simulink model "atrias_system_1khz"  (R2016b)
settings: Solver=FixedStepDiscrete  StartTime=0.0  StopTime=inf  FixedStep=sample_time  RelTol=1e-3
undefined symbols (not defined in the file or in its folder): gui_disable_cmd, gui_enable_cmd, gui_exit_cmd, gui_reset_cmd, HARD_MOTOR_POSITION_LIMITS_LOWER, HARD_MOTOR_POSITION_LIMITS_UPPER, HIP_ABS_MAX_ENCODER_TICKS, HIP_CURRENT_LIMIT, HIP_INC_MAX_ENCODER_TICKS, HIP_MOTOR_CONSTANT, HIP_MTR_GEAR_RATIO, HIP_MTR_MAX_TORQUE, LEFT_MOTOR_HIP_DIRECTION, LEG1_MOTOR_A_DIRECTION, LEG1_MOTOR_B_DIRECTION, LEG2_MOTOR_A_DIRECTION, LEG2_MOTOR_B_DIRECTION, LEG_CURRENT_LIMIT, LEG_INC_ENCODER_DIRECTION_LEFT_BACK, LEG_INC_ENCODER_DIRECTION_LEFT_FRONT, LEG_INC_ENCODER_DIRECTION_RIGHT_BACK, LEG_INC_ENCODER_DIRECTION_RIGHT_FRONT, LEG_INC_ENCODER_RAD_PER_TICK, LEG_MOTOR_CONSTANT, LEG_MTR_GEAR_RATIO, LEG_MTR_MAX_TORQUE, max_hip_velocity, max_motor_velocity, MEDULLA_ADC_MAX_VOLTS, MEDULLA_ADC_OFFSET_COUNTS, MEDULLA_STATE_ERROR, MEDULLA_STATE_HALT, MEDULLA_STATE_IDLE, MEDULLA_STATE_RESET, MEDULLA_STATE_RUN, MOTOR_POSITION_LIMITS_LOWER, MOTOR_POSITION_LIMITS_UPPER, MTR_HIP_MAX_CURRENT, MTR_MAX_CONT_CURRENT, MTR_MAX_COUNT, MTR_MAX_CURRENT, MTR_MAX_TEMP, RIGHT_MOTOR_HIP_DIRECTION
libraries: xpcethercatlib x190, simulink x37
(part 3 of 4)

== system atrias_system_1khz/DAQ/Conversion ==
  note: Convert from Current to Torque
  Elmo Current : Inport
  Constant10 : Constant  Value=LEG_MOTOR_CONSTANT
  Constant11 : Constant  Value=LEG_MTR_GEAR_RATIO
  Convert Elmo PDO to Current : Gain  Gain=MTR_MAX_CONT_CURRENT/1000
  Divide2 : Product  Inputs=****
  LEG1_MOTOR_A_DIRECTION : Constant  Value=LEG1_MOTOR_A_DIRECTION
  LEG1_MOTOR_B_DIRECTION : Constant  Value=LEG1_MOTOR_B_DIRECTION
  LEG2_MOTOR_A_DIRECTION : Constant  Value=LEG2_MOTOR_A_DIRECTION
  LEG2_MOTOR_B_DIRECTION : Constant  Value=LEG2_MOTOR_B_DIRECTION
  Mux2 : Mux
  Torque : Outport
  wires:
  Elmo Current/1 -> Convert Elmo PDO to Current/1
  Constant11/1 -> Divide2/2
  Convert Elmo PDO to Current/1 -> Divide2/3
  Constant10/1 -> Divide2/1
  Divide2/1 -> Torque/1
  LEG1_MOTOR_A_DIRECTION/1 -> Mux2/1
  LEG2_MOTOR_B_DIRECTION/1 -> Mux2/4
  Mux2/1 -> Divide2/4
  LEG2_MOTOR_A_DIRECTION/1 -> Mux2/3
  LEG1_MOTOR_B_DIRECTION/1 -> Mux2/2

== system atrias_system_1khz/DAQ/Conversion1 ==
  note: Convert from Current to Torque
  Elmo Current : Inport
  Constant10 : Constant  Value=LEG_MOTOR_CONSTANT
  Constant11 : Constant  Value=LEG_MTR_GEAR_RATIO
  Convert Elmo PDO to Current : Gain  Gain=MTR_MAX_CONT_CURRENT/1000
  Divide2 : Product  Inputs=****
  LEG1_MOTOR_A_DIRECTION : Constant  Value=LEG1_MOTOR_A_DIRECTION
  LEG1_MOTOR_B_DIRECTION : Constant  Value=LEG1_MOTOR_B_DIRECTION
  LEG2_MOTOR_A_DIRECTION : Constant  Value=LEG2_MOTOR_A_DIRECTION
  LEG2_MOTOR_B_DIRECTION : Constant  Value=LEG2_MOTOR_B_DIRECTION
  Mux2 : Mux
  Torque : Outport
  wires:
  LEG1_MOTOR_B_DIRECTION/1 -> Mux2/2
  LEG2_MOTOR_A_DIRECTION/1 -> Mux2/3
  Mux2/1 -> Divide2/4
  LEG2_MOTOR_B_DIRECTION/1 -> Mux2/4
  LEG1_MOTOR_A_DIRECTION/1 -> Mux2/1
  Divide2/1 -> Torque/1
  Constant10/1 -> Divide2/1
  Convert Elmo PDO to Current/1 -> Divide2/3
  Constant11/1 -> Divide2/2
  Elmo Current/1 -> Convert Elmo PDO to Current/1

== system atrias_system_1khz/DAQ/Convert geared rad//s to rotor cnts//s ==
  in : Inport
  Gear Ratio : Gain  Gain=LEG_MTR_GEAR_RATIO
  LEG1_MOTOR_A_DIRECTION : Constant  Value=LEG1_MOTOR_A_DIRECTION
  LEG1_MOTOR_B_DIRECTION : Constant  Value=LEG1_MOTOR_B_DIRECTION
  LEG2_MOTOR_A_DIRECTION : Constant  Value=LEG2_MOTOR_A_DIRECTION
  LEG2_MOTOR_B_DIRECTION : Constant  Value=LEG2_MOTOR_B_DIRECTION
  Mux2 : Mux
  Product : Product  RndMeth=Zero
  RadPerSecToCountsPerSec : Gain  Gain=14000/(2*pi)
  out : Outport
  wires:
  RadPerSecToCountsPerSec/1 -> Gear Ratio/1
  in/1 -> RadPerSecToCountsPerSec/1
  LEG1_MOTOR_A_DIRECTION/1 -> Mux2/1
  Product/1 -> out/1
  Gear Ratio/1 -> Product/1
  LEG2_MOTOR_B_DIRECTION/1 -> Mux2/4
  Mux2/1 -> Product/2
  LEG2_MOTOR_A_DIRECTION/1 -> Mux2/3
  LEG1_MOTOR_B_DIRECTION/1 -> Mux2/2

== system atrias_system_1khz/DAQ/Convert rotor cnt//s to geared rad//s ==
  in : Inport
  Divide : Product  Inputs=*//
  Gear Ratio : Gain  Gain=LEG_MTR_GEAR_RATIO
  LEG1_MOTOR_A_DIRECTION : Constant  Value=LEG1_MOTOR_A_DIRECTION
  LEG1_MOTOR_B_DIRECTION : Constant  Value=LEG1_MOTOR_B_DIRECTION
  LEG2_MOTOR_A_DIRECTION : Constant  Value=LEG2_MOTOR_A_DIRECTION
  LEG2_MOTOR_B_DIRECTION : Constant  Value=LEG2_MOTOR_B_DIRECTION
  Mux : Mux  Inputs=2
  Mux2 : Mux
  RadPerSecToCountsPerSec : Constant  Value=14000/(2*pi)
  out : Outport
  wires:
  RadPerSecToCountsPerSec/1 -> Gear Ratio/1
  in/1 -> Divide/1
  LEG1_MOTOR_A_DIRECTION/1 -> Mux2/1
  Divide/1 -> out/1
  Gear Ratio/1 -> Divide/2
  LEG2_MOTOR_B_DIRECTION/1 -> Mux2/4
  Mux2/1 -> Mux/1, Mux/2
  LEG2_MOTOR_A_DIRECTION/1 -> Mux2/3
  LEG1_MOTOR_B_DIRECTION/1 -> Mux2/2
  Mux/1 -> Divide/3

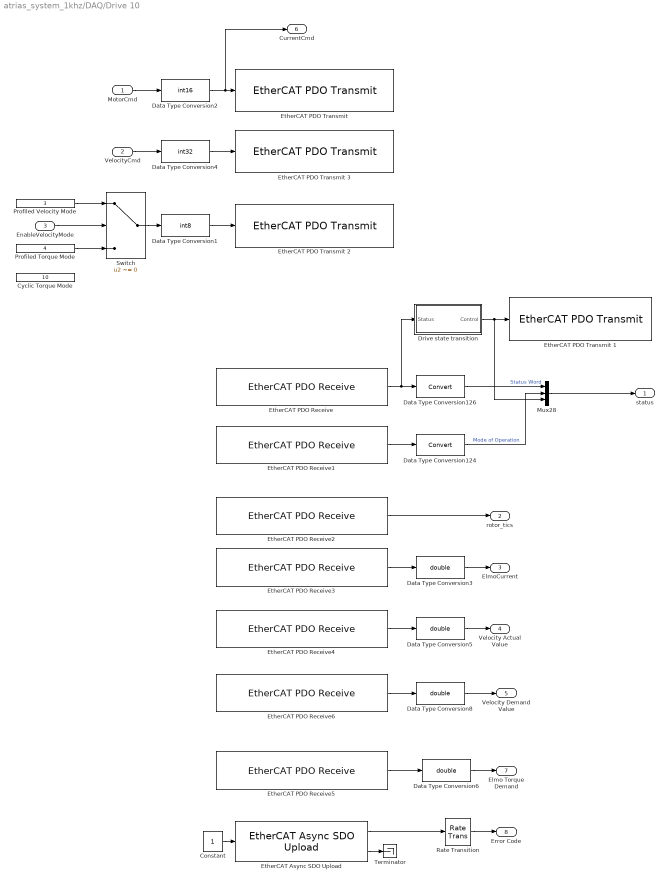
== system atrias_system_1khz/DAQ/Drive 10 ==
  MotorCmd : Inport
  VelocityCmd : Inport  Port=2
  EnableVelocityMode : Inport  Port=3
  Constant : Constant  OutDataTypeStr=int32
  Cyclic Torque Mode : Constant  Value=10  OutDataTypeStr=Inherit: Inherit via back propagation
  Data Type Conversion1 : DataTypeConversion  OutDataTypeStr=int8
  Data Type Conversion124 : DataTypeConversion
  Data Type Conversion126 : DataTypeConversion
  Data Type Conversion2 : DataTypeConversion  OutDataTypeStr=int16
  Data Type Conversion{3,5..6,8} (4 alike) : DataTypeConversion  OutDataTypeStr=double
  Data Type Conversion4 : DataTypeConversion  OutDataTypeStr=int32
  Drive state transition : Subsystem
  EtherCAT Async SDO Upload : xpcethercatlib/EtherCAT Async SDO Upload  index=24639  subIndex=0  sig_type=uint16  sig_dim=1  device_id=0  slave_name=Drive 10 (Elmo Drive)  sample_time=0.100  slave_addr=1010  selected_slave=Term 1 (EK1100)  timeout=500  slave_found=1
  EtherCAT PDO Receive : xpcethercatlib/EtherCAT PDO Receive  Priority=2  sig_name=Drive 10 (Elmo Drive).Inputs.Status word  sig_offset=3296  sig_type=uint16  type_size=16  sig_dim=1  device_id=0  sample_time=0.001000
  EtherCAT PDO Receive1 : xpcethercatlib/EtherCAT PDO Receive  Priority=2  sig_name=Drive 10 (Elmo Drive).Inputs.Mode of operation display  sig_offset=3312  sig_type=int8  type_size=8  sig_dim=1  device_id=0  sample_time=0.001000
  EtherCAT PDO Receive2 : xpcethercatlib/EtherCAT PDO Receive  Priority=2  sig_name=Drive 10 (Elmo Drive).Inputs.Position actual value  sig_offset=3328  sig_type=int32  type_size=32  sig_dim=1  device_id=0  sample_time=0.001000
  EtherCAT PDO Receive3 : xpcethercatlib/EtherCAT PDO Receive  Priority=2  sig_name=Drive 10 (Elmo Drive).Inputs.Current actual value  sig_offset=3440  sig_type=int16  type_size=16  sig_dim=1  device_id=0  sample_time=0.001000
  EtherCAT PDO Receive4 : xpcethercatlib/EtherCAT PDO Receive  Priority=2  sig_name=Drive 10 (Elmo Drive).Inputs.Velocity actual value  sig_offset=3392  sig_type=int32  type_size=32  sig_dim=1  device_id=0  sample_time=0.001000
  EtherCAT PDO Receive5 : xpcethercatlib/EtherCAT PDO Receive  Priority=2  sig_name=Drive 10 (Elmo Drive).Inputs.Torque demand value  sig_offset=3424  sig_type=int16  type_size=16  sig_dim=1  device_id=0  sample_time=0.001000
  EtherCAT PDO Receive6 : xpcethercatlib/EtherCAT PDO Receive  Priority=2  sig_name=Drive 10 (Elmo Drive).Inputs.Velocity demand [cnt/sec]  sig_offset=3360  sig_type=int32  type_size=32  sig_dim=1  device_id=0  sample_time=0.001000
  "EtherCAT PDO Transmit " : xpcethercatlib/EtherCAT PDO Transmit   Priority=3  sig_name=Drive 10 (Elmo Drive).Outputs.Target Torque  sig_offset=3328  sig_type=int16  type_size=16  sig_dim=1  device_id=0  sample_time=0.001000
  EtherCAT PDO Transmit 1 : xpcethercatlib/EtherCAT PDO Transmit   Priority=3  sig_name=Drive 10 (Elmo Drive).Outputs.Control word  sig_offset=3296  sig_type=uint16  type_size=16  sig_dim=1  device_id=0  sample_time=0.001000
  EtherCAT PDO Transmit 2 : xpcethercatlib/EtherCAT PDO Transmit   Priority=3  sig_name=Drive 10 (Elmo Drive).Outputs.Mode of operation  sig_offset=3312  sig_type=int8  type_size=8  sig_dim=1  device_id=0  sample_time=0.001000
  EtherCAT PDO Transmit 3 : xpcethercatlib/EtherCAT PDO Transmit   Priority=3  sig_name=Drive 10 (Elmo Drive).Outputs.Target Velocity  sig_offset=3360  sig_type=int32  type_size=32  sig_dim=1  device_id=0  sample_time=0.001000
  Mux28 : Mux  Inputs=3
  Profiled Torque Mode : Constant  Value=4  OutDataTypeStr=Inherit: Inherit via back propagation
  Profiled Velocity Mode : Constant  Value=3  OutDataTypeStr=Inherit: Inherit via back propagation
  Rate Transition : RateTransition  Deterministic=off  OutPortSampleTime=sample_time
  Switch : Switch  Criteria=u2 ~= 0
  Terminator : Terminator
  status : Outport
  rotor_tics : Outport  Port=2
  ElmoCurrent : Outport  Port=3
  Velocity Actual Value : Outport  Port=4
  Velocity Demand Value : Outport  Port=5
  CurrentCmd : Outport  Port=6
  Elmo Torque Demand : Outport  Port=7
  Error Code : Outport  Port=8
  wires:
  Data Type Conversion3/1 -> ElmoCurrent/1
  EtherCAT PDO Receive3/1 -> Data Type Conversion3/1
  EtherCAT PDO Receive2/1 -> rotor_tics/1
  Data Type Conversion2/1 -> CurrentCmd/1, "EtherCAT PDO Transmit "/1
  MotorCmd/1 -> Data Type Conversion2/1
  Data Type Conversion1/1 -> EtherCAT PDO Transmit 2/1
  Drive state transition/1(Control) -> EtherCAT PDO Transmit 1/1, Mux28/3
  Switch/1 -> Data Type Conversion1/1
  Data Type Conversion124/1 -> Mux28/2  "Mode of Operation"
  Data Type Conversion126/1 -> Mux28/1  "Status Word"
  Mux28/1 -> status/1
  EtherCAT PDO Receive1/1 -> Data Type Conversion124/1
  EtherCAT PDO Receive/1 -> Drive state transition/1(Status), Data Type Conversion126/1
  Profiled Torque Mode/1 -> Switch/3
  Profiled Velocity Mode/1 -> Switch/1
  EnableVelocityMode/1 -> Switch/2
  Data Type Conversion4/1 -> EtherCAT PDO Transmit 3/1
  VelocityCmd/1 -> Data Type Conversion4/1
  EtherCAT PDO Receive4/1 -> Data Type Conversion5/1
  Data Type Conversion5/1 -> Velocity Actual Value/1
  Data Type Conversion6/1 -> Elmo Torque Demand/1
  EtherCAT PDO Receive5/1 -> Data Type Conversion6/1
  EtherCAT Async SDO Upload/1 -> Rate Transition/1
  Constant/1 -> EtherCAT Async SDO Upload/1
  Rate Transition/1 -> Error Code/1
  EtherCAT Async SDO Upload/2 -> Terminator/1
  EtherCAT PDO Receive6/1 -> Data Type Conversion8/1
  Data Type Conversion8/1 -> Velocity Demand Value/1

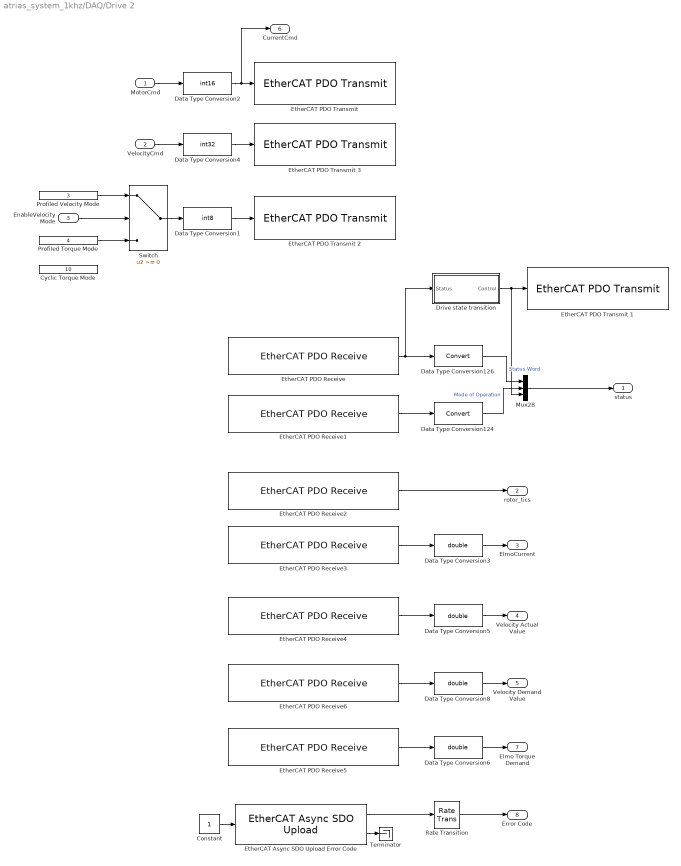
== system atrias_system_1khz/DAQ/Drive 2 ==
  MotorCmd : Inport
  VelocityCmd : Inport  Port=2
  EnableVelocity Mode : Inport  Port=3
  Constant : Constant  OutDataTypeStr=int32
  Cyclic Torque Mode : Constant  Value=10  OutDataTypeStr=Inherit: Inherit via back propagation
  Data Type Conversion1 : DataTypeConversion  OutDataTypeStr=int8
  Data Type Conversion124 : DataTypeConversion
  Data Type Conversion126 : DataTypeConversion
  Data Type Conversion2 : DataTypeConversion  OutDataTypeStr=int16
  Data Type Conversion{3,5..6,8} (4 alike) : DataTypeConversion  OutDataTypeStr=double
  Data Type Conversion4 : DataTypeConversion  OutDataTypeStr=int32
  Drive state transition : Subsystem
  EtherCAT Async SDO Upload Error Code : xpcethercatlib/EtherCAT Async SDO Upload  index=24639  subIndex=0  sig_type=uint16  sig_dim=1  device_id=0  slave_name=Box 2 (Elmo Drive)  sample_time=0.100  slave_addr=1002  selected_slave=Term 1 (EK1100)  timeout=500  slave_found=1
  EtherCAT PDO Receive : xpcethercatlib/EtherCAT PDO Receive  Priority=2  sig_name=Box 2 (Elmo Drive).Inputs.Status word  sig_offset=2816  sig_type=uint16  type_size=16  sig_dim=1  device_id=0  sample_time=0.001000
  EtherCAT PDO Receive1 : xpcethercatlib/EtherCAT PDO Receive  Priority=2  sig_name=Box 2 (Elmo Drive).Inputs.Mode of operation display  sig_offset=2832  sig_type=int8  type_size=8  sig_dim=1  device_id=0  sample_time=0.001000
  EtherCAT PDO Receive2 : xpcethercatlib/EtherCAT PDO Receive  Priority=2  sig_name=Box 2 (Elmo Drive).Inputs.Position actual value  sig_offset=2848  sig_type=int32  type_size=32  sig_dim=1  device_id=0  sample_time=0.001000
  EtherCAT PDO Receive3 : xpcethercatlib/EtherCAT PDO Receive  Priority=2  sig_name=Box 2 (Elmo Drive).Inputs.Current actual value  sig_offset=2960  sig_type=int16  type_size=16  sig_dim=1  device_id=0  sample_time=0.001000
  EtherCAT PDO Receive4 : xpcethercatlib/EtherCAT PDO Receive  Priority=2  sig_name=Box 2 (Elmo Drive).Inputs.Velocity actual value  sig_offset=2912  sig_type=int32  type_size=32  sig_dim=1  device_id=0  sample_time=0.001000
  EtherCAT PDO Receive5 : xpcethercatlib/EtherCAT PDO Receive  Priority=2  sig_name=Box 2 (Elmo Drive).Inputs.Torque demand value  sig_offset=2944  sig_type=int16  type_size=16  sig_dim=1  device_id=0  sample_time=0.001000
  EtherCAT PDO Receive6 : xpcethercatlib/EtherCAT PDO Receive  Priority=2  sig_name=Box 2 (Elmo Drive).Inputs.Velocity demand [cnt/sec]  sig_offset=2880  sig_type=int32  type_size=32  sig_dim=1  device_id=0  sample_time=0.001000
  "EtherCAT PDO Transmit " : xpcethercatlib/EtherCAT PDO Transmit   Priority=3  sig_name=Box 2 (Elmo Drive).Outputs.Target Torque  sig_offset=2848  sig_type=int16  type_size=16  sig_dim=1  device_id=0  sample_time=0.001000
  EtherCAT PDO Transmit 1 : xpcethercatlib/EtherCAT PDO Transmit   Priority=3  sig_name=Box 2 (Elmo Drive).Outputs.Control word  sig_offset=2816  sig_type=uint16  type_size=16  sig_dim=1  device_id=0  sample_time=0.001000
  EtherCAT PDO Transmit 2 : xpcethercatlib/EtherCAT PDO Transmit   Priority=3  sig_name=Box 2 (Elmo Drive).Outputs.Mode of operation  sig_offset=2832  sig_type=int8  type_size=8  sig_dim=1  device_id=0  sample_time=0.001000
  EtherCAT PDO Transmit 3 : xpcethercatlib/EtherCAT PDO Transmit   Priority=3  sig_name=Box 2 (Elmo Drive).Outputs.Target Velocity  sig_offset=2880  sig_type=int32  type_size=32  sig_dim=1  device_id=0  sample_time=0.001000
  Mux28 : Mux  Inputs=3
  Profiled Torque Mode : Constant  Value=4  OutDataTypeStr=Inherit: Inherit via back propagation
  Profiled Velocity Mode : Constant  Value=3  OutDataTypeStr=Inherit: Inherit via back propagation
  Rate Transition : RateTransition  Deterministic=off  OutPortSampleTime=sample_time
  Switch : Switch  Criteria=u2 ~= 0
  Terminator : Terminator
  status : Outport
  rotor_tics : Outport  Port=2
  ElmoCurrent : Outport  Port=3
  Velocity Actual Value : Outport  Port=4
  Velocity Demand Value : Outport  Port=5
  CurrentCmd : Outport  Port=6
  Elmo Torque Demand : Outport  Port=7
  Error Code : Outport  Port=8
  wires:
  EtherCAT PDO Receive1/1 -> Data Type Conversion124/1
  Mux28/1 -> status/1
  Data Type Conversion126/1 -> Mux28/1  "Status Word"
  Data Type Conversion124/1 -> Mux28/2  "Mode of Operation"
  Drive state transition/1(Control) -> Mux28/3, EtherCAT PDO Transmit 1/1
  EtherCAT PDO Receive2/1 -> rotor_tics/1
  EtherCAT PDO Receive3/1 -> Data Type Conversion3/1
  Data Type Conversion3/1 -> ElmoCurrent/1
  Data Type Conversion2/1 -> CurrentCmd/1, "EtherCAT PDO Transmit "/1
  MotorCmd/1 -> Data Type Conversion2/1
  Data Type Conversion1/1 -> EtherCAT PDO Transmit 2/1
  Switch/1 -> Data Type Conversion1/1
  Profiled Torque Mode/1 -> Switch/3
  Profiled Velocity Mode/1 -> Switch/1
  EnableVelocity Mode/1 -> Switch/2
  VelocityCmd/1 -> Data Type Conversion4/1
  Data Type Conversion4/1 -> EtherCAT PDO Transmit 3/1
  EtherCAT PDO Receive4/1 -> Data Type Conversion5/1
  Data Type Conversion5/1 -> Velocity Actual Value/1
  EtherCAT PDO Receive/1 -> Data Type Conversion126/1, Drive state transition/1(Status)
  Data Type Conversion6/1 -> Elmo Torque Demand/1
  EtherCAT PDO Receive5/1 -> Data Type Conversion6/1
  EtherCAT Async SDO Upload Error Code/1 -> Rate Transition/1
  Constant/1 -> EtherCAT Async SDO Upload Error Code/1
  Rate Transition/1 -> Error Code/1
  EtherCAT Async SDO Upload Error Code/2 -> Terminator/1
  EtherCAT PDO Receive6/1 -> Data Type Conversion8/1
  Data Type Conversion8/1 -> Velocity Demand Value/1

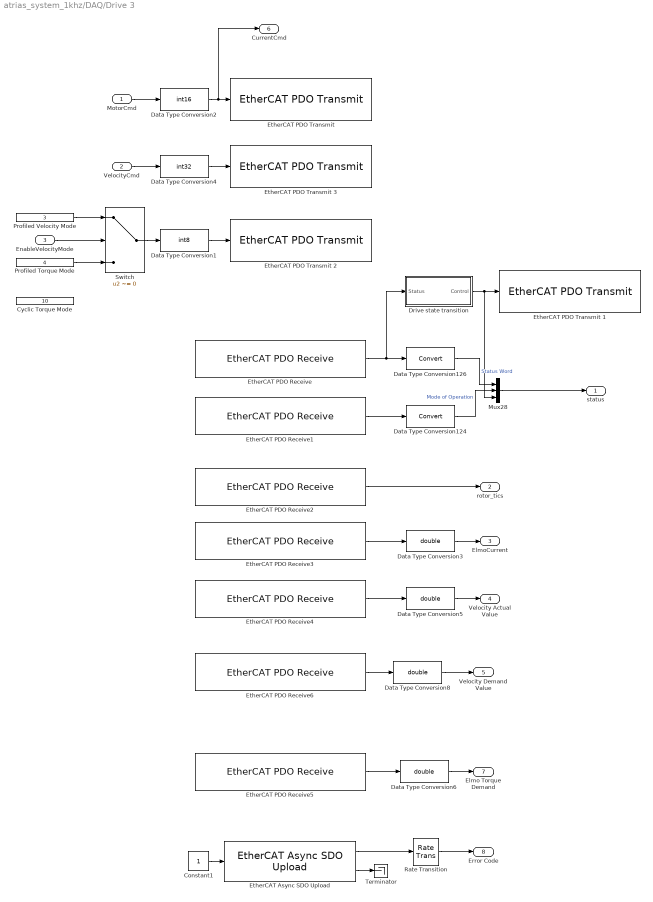
== system atrias_system_1khz/DAQ/Drive 3 ==
  MotorCmd : Inport
  VelocityCmd : Inport  Port=2
  EnableVelocityMode : Inport  Port=3
  Constant1 : Constant  OutDataTypeStr=int32
  Cyclic Torque Mode : Constant  Value=10  OutDataTypeStr=Inherit: Inherit via back propagation
  Data Type Conversion1 : DataTypeConversion  OutDataTypeStr=int8
  Data Type Conversion124 : DataTypeConversion
  Data Type Conversion126 : DataTypeConversion
  Data Type Conversion2 : DataTypeConversion  OutDataTypeStr=int16
  Data Type Conversion{3,5..6,8} (4 alike) : DataTypeConversion  OutDataTypeStr=double
  Data Type Conversion4 : DataTypeConversion  OutDataTypeStr=int32
  Drive state transition : Subsystem
  EtherCAT Async SDO Upload : xpcethercatlib/EtherCAT Async SDO Upload  index=24639  subIndex=0  sig_type=uint16  sig_dim=1  device_id=0  slave_name=Box 3 (Elmo Drive)  sample_time=0.100  slave_addr=1003  selected_slave=Term 1 (EK1100)  timeout=500  slave_found=1
  EtherCAT PDO Receive : xpcethercatlib/EtherCAT PDO Receive  Priority=2  sig_name=Box 3 (Elmo Drive).Inputs.Status word  sig_offset=2976  sig_type=uint16  type_size=16  sig_dim=1  device_id=0  sample_time=0.001000
  EtherCAT PDO Receive1 : xpcethercatlib/EtherCAT PDO Receive  Priority=2  sig_name=Box 3 (Elmo Drive).Inputs.Mode of operation display  sig_offset=2992  sig_type=int8  type_size=8  sig_dim=1  device_id=0  sample_time=0.001000
  EtherCAT PDO Receive2 : xpcethercatlib/EtherCAT PDO Receive  Priority=2  sig_name=Box 3 (Elmo Drive).Inputs.Position actual value  sig_offset=3008  sig_type=int32  type_size=32  sig_dim=1  device_id=0  sample_time=0.001000
  EtherCAT PDO Receive3 : xpcethercatlib/EtherCAT PDO Receive  Priority=2  sig_name=Box 3 (Elmo Drive).Inputs.Current actual value  sig_offset=3120  sig_type=int16  type_size=16  sig_dim=1  device_id=0  sample_time=0.001000
  EtherCAT PDO Receive4 : xpcethercatlib/EtherCAT PDO Receive  Priority=2  sig_name=Box 3 (Elmo Drive).Inputs.Velocity actual value  sig_offset=3072  sig_type=int32  type_size=32  sig_dim=1  device_id=0  sample_time=0.001000
  EtherCAT PDO Receive5 : xpcethercatlib/EtherCAT PDO Receive  Priority=2  sig_name=Box 3 (Elmo Drive).Inputs.Torque demand value  sig_offset=3104  sig_type=int16  type_size=16  sig_dim=1  device_id=0  sample_time=0.001000
  EtherCAT PDO Receive6 : xpcethercatlib/EtherCAT PDO Receive  Priority=2  sig_name=Box 3 (Elmo Drive).Inputs.Velocity demand [cnt/sec]  sig_offset=3040  sig_type=int32  type_size=32  sig_dim=1  device_id=0  sample_time=0.001000
  "EtherCAT PDO Transmit " : xpcethercatlib/EtherCAT PDO Transmit   Priority=3  sig_name=Box 3 (Elmo Drive).Outputs.Target Torque  sig_offset=3008  sig_type=int16  type_size=16  sig_dim=1  device_id=0  sample_time=0.001000
  EtherCAT PDO Transmit 1 : xpcethercatlib/EtherCAT PDO Transmit   Priority=3  sig_name=Box 3 (Elmo Drive).Outputs.Control word  sig_offset=2976  sig_type=uint16  type_size=16  sig_dim=1  device_id=0  sample_time=0.001000
  EtherCAT PDO Transmit 2 : xpcethercatlib/EtherCAT PDO Transmit   Priority=3  sig_name=Box 3 (Elmo Drive).Outputs.Mode of operation  sig_offset=2992  sig_type=int8  type_size=8  sig_dim=1  device_id=0  sample_time=0.001000
  EtherCAT PDO Transmit 3 : xpcethercatlib/EtherCAT PDO Transmit   Priority=3  sig_name=Box 3 (Elmo Drive).Outputs.Target Velocity  sig_offset=3040  sig_type=int32  type_size=32  sig_dim=1  device_id=0  sample_time=0.001000
  Mux28 : Mux  Inputs=3
  Profiled Torque Mode : Constant  Value=4  OutDataTypeStr=Inherit: Inherit via back propagation
  Profiled Velocity Mode : Constant  Value=3  OutDataTypeStr=Inherit: Inherit via back propagation
  Rate Transition : RateTransition  Deterministic=off  OutPortSampleTime=sample_time
  Switch : Switch  Criteria=u2 ~= 0
  Terminator : Terminator
  status : Outport
  rotor_tics : Outport  Port=2
  ElmoCurrent : Outport  Port=3
  Velocity Actual Value : Outport  Port=4
  Velocity Demand Value : Outport  Port=5
  CurrentCmd : Outport  Port=6
  Elmo Torque Demand : Outport  Port=7
  Error Code : Outport  Port=8
  wires:
  EtherCAT PDO Receive1/1 -> Data Type Conversion124/1
  Mux28/1 -> status/1
  Data Type Conversion126/1 -> Mux28/1  "Status Word"
  Data Type Conversion124/1 -> Mux28/2  "Mode of Operation"
  Drive state transition/1(Control) -> Mux28/3, EtherCAT PDO Transmit 1/1
  EtherCAT PDO Receive2/1 -> rotor_tics/1
  EtherCAT PDO Receive3/1 -> Data Type Conversion3/1
  Data Type Conversion3/1 -> ElmoCurrent/1
  Data Type Conversion2/1 -> CurrentCmd/1, "EtherCAT PDO Transmit "/1
  MotorCmd/1 -> Data Type Conversion2/1
  Data Type Conversion1/1 -> EtherCAT PDO Transmit 2/1
  Switch/1 -> Data Type Conversion1/1
  Profiled Torque Mode/1 -> Switch/3
  Profiled Velocity Mode/1 -> Switch/1
  EnableVelocityMode/1 -> Switch/2
  VelocityCmd/1 -> Data Type Conversion4/1
  Data Type Conversion4/1 -> EtherCAT PDO Transmit 3/1
  EtherCAT PDO Receive4/1 -> Data Type Conversion5/1
  Data Type Conversion5/1 -> Velocity Actual Value/1
  EtherCAT PDO Receive/1 -> Data Type Conversion126/1, Drive state transition/1(Status)
  Data Type Conversion6/1 -> Elmo Torque Demand/1
  EtherCAT PDO Receive5/1 -> Data Type Conversion6/1
  EtherCAT Async SDO Upload/1 -> Rate Transition/1
  Constant1/1 -> EtherCAT Async SDO Upload/1
  Rate Transition/1 -> Error Code/1
  EtherCAT Async SDO Upload/2 -> Terminator/1
  EtherCAT PDO Receive6/1 -> Data Type Conversion8/1
  Data Type Conversion8/1 -> Velocity Demand Value/1

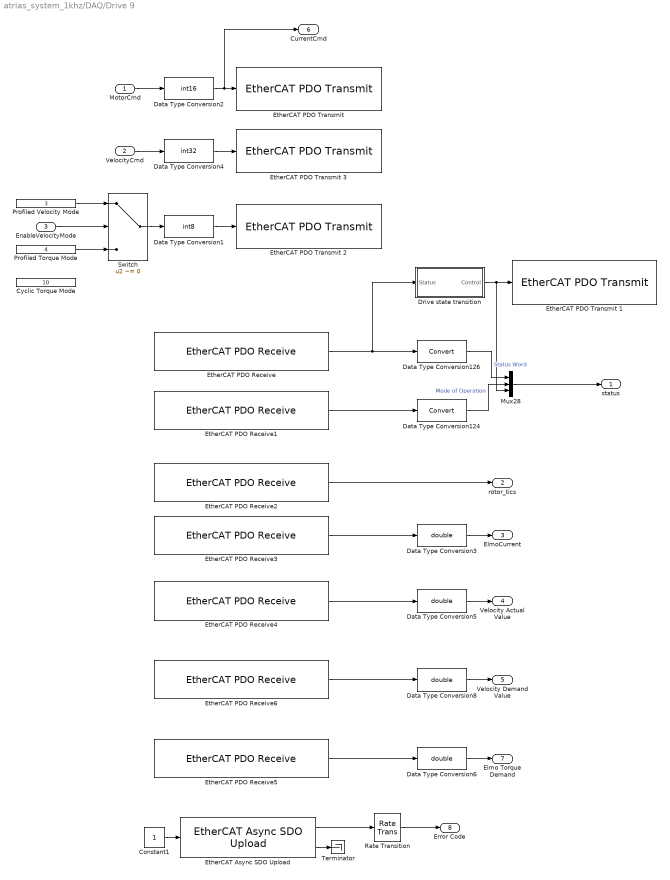
== system atrias_system_1khz/DAQ/Drive 9 ==
  MotorCmd : Inport
  VelocityCmd : Inport  Port=2
  EnableVelocityMode : Inport  Port=3
  Constant1 : Constant  OutDataTypeStr=int32
  Cyclic Torque Mode : Constant  Value=10  OutDataTypeStr=Inherit: Inherit via back propagation
  Data Type Conversion1 : DataTypeConversion  OutDataTypeStr=int8
  Data Type Conversion124 : DataTypeConversion
  Data Type Conversion126 : DataTypeConversion
  Data Type Conversion2 : DataTypeConversion  OutDataTypeStr=int16
  Data Type Conversion{3,5..6,8} (4 alike) : DataTypeConversion  OutDataTypeStr=double
  Data Type Conversion4 : DataTypeConversion  OutDataTypeStr=int32
  Drive state transition : Subsystem
  EtherCAT Async SDO Upload : xpcethercatlib/EtherCAT Async SDO Upload  index=24639  subIndex=0  sig_type=uint16  sig_dim=1  device_id=0  slave_name=Drive 9 (Elmo Drive)  sample_time=0.100  slave_addr=1009  selected_slave=Term 1 (EK1100)  timeout=500  slave_found=1
  EtherCAT PDO Receive : xpcethercatlib/EtherCAT PDO Receive  Priority=2  sig_name=Drive 9 (Elmo Drive).Inputs.Status word  sig_offset=3136  sig_type=uint16  type_size=16  sig_dim=1  device_id=0  sample_time=0.001000
  EtherCAT PDO Receive1 : xpcethercatlib/EtherCAT PDO Receive  Priority=2  sig_name=Drive 9 (Elmo Drive).Inputs.Mode of operation display  sig_offset=3152  sig_type=int8  type_size=8  sig_dim=1  device_id=0  sample_time=0.001000
  EtherCAT PDO Receive2 : xpcethercatlib/EtherCAT PDO Receive  Priority=2  sig_name=Drive 9 (Elmo Drive).Inputs.Position actual value  sig_offset=3168  sig_type=int32  type_size=32  sig_dim=1  device_id=0  sample_time=0.001000
  EtherCAT PDO Receive3 : xpcethercatlib/EtherCAT PDO Receive  Priority=2  sig_name=Drive 9 (Elmo Drive).Inputs.Current actual value  sig_offset=3280  sig_type=int16  type_size=16  sig_dim=1  device_id=0  sample_time=0.001000
  EtherCAT PDO Receive4 : xpcethercatlib/EtherCAT PDO Receive  Priority=2  sig_name=Drive 9 (Elmo Drive).Inputs.Velocity actual value  sig_offset=3232  sig_type=int32  type_size=32  sig_dim=1  device_id=0  sample_time=0.001000
  EtherCAT PDO Receive5 : xpcethercatlib/EtherCAT PDO Receive  Priority=2  sig_name=Drive 9 (Elmo Drive).Inputs.Torque demand value  sig_offset=3264  sig_type=int16  type_size=16  sig_dim=1  device_id=0  sample_time=0.001000
  EtherCAT PDO Receive6 : xpcethercatlib/EtherCAT PDO Receive  Priority=2  sig_name=Drive 9 (Elmo Drive).Inputs.Velocity demand [cnt/sec]  sig_offset=3200  sig_type=int32  type_size=32  sig_dim=1  device_id=0  sample_time=0.001000
  "EtherCAT PDO Transmit " : xpcethercatlib/EtherCAT PDO Transmit   Priority=3  sig_name=Drive 9 (Elmo Drive).Outputs.Target Torque  sig_offset=3168  sig_type=int16  type_size=16  sig_dim=1  device_id=0  sample_time=0.001000
  EtherCAT PDO Transmit 1 : xpcethercatlib/EtherCAT PDO Transmit   Priority=3  sig_name=Drive 9 (Elmo Drive).Outputs.Control word  sig_offset=3136  sig_type=uint16  type_size=16  sig_dim=1  device_id=0  sample_time=0.001000
  EtherCAT PDO Transmit 2 : xpcethercatlib/EtherCAT PDO Transmit   Priority=3  sig_name=Drive 9 (Elmo Drive).Outputs.Mode of operation  sig_offset=3152  sig_type=int8  type_size=8  sig_dim=1  device_id=0  sample_time=0.001000
  EtherCAT PDO Transmit 3 : xpcethercatlib/EtherCAT PDO Transmit   Priority=3  sig_name=Drive 9 (Elmo Drive).Outputs.Target Velocity  sig_offset=3200  sig_type=int32  type_size=32  sig_dim=1  device_id=0  sample_time=0.001000
  Mux28 : Mux  Inputs=3
  Profiled Torque Mode : Constant  Value=4  OutDataTypeStr=Inherit: Inherit via back propagation
  Profiled Velocity Mode : Constant  Value=3  OutDataTypeStr=Inherit: Inherit via back propagation
  Rate Transition : RateTransition  Deterministic=off  OutPortSampleTime=sample_time
  Switch : Switch  Criteria=u2 ~= 0
  Terminator : Terminator
  status : Outport
  rotor_tics : Outport  Port=2
  ElmoCurrent : Outport  Port=3
  Velocity Actual Value : Outport  Port=4
  Velocity Demand Value : Outport  Port=5
  CurrentCmd : Outport  Port=6
  Elmo Torque Demand : Outport  Port=7
  Error Code : Outport  Port=8
  wires:
  EtherCAT PDO Receive/1 -> Drive state transition/1(Status), Data Type Conversion126/1
  EtherCAT PDO Receive1/1 -> Data Type Conversion124/1
  Mux28/1 -> status/1
  Data Type Conversion126/1 -> Mux28/1  "Status Word"
  Data Type Conversion124/1 -> Mux28/2  "Mode of Operation"
  Drive state transition/1(Control) -> Mux28/3, EtherCAT PDO Transmit 1/1
  EtherCAT PDO Receive2/1 -> rotor_tics/1
  EtherCAT PDO Receive3/1 -> Data Type Conversion3/1
  Data Type Conversion3/1 -> ElmoCurrent/1
  Data Type Conversion2/1 -> CurrentCmd/1, "EtherCAT PDO Transmit "/1
  MotorCmd/1 -> Data Type Conversion2/1
  Data Type Conversion1/1 -> EtherCAT PDO Transmit 2/1
  Switch/1 -> Data Type Conversion1/1
  Profiled Torque Mode/1 -> Switch/3
  Profiled Velocity Mode/1 -> Switch/1
  EnableVelocityMode/1 -> Switch/2
  Data Type Conversion4/1 -> EtherCAT PDO Transmit 3/1
  VelocityCmd/1 -> Data Type Conversion4/1
  EtherCAT PDO Receive4/1 -> Data Type Conversion5/1
  Data Type Conversion5/1 -> Velocity Actual Value/1
  Data Type Conversion6/1 -> Elmo Torque Demand/1
  EtherCAT PDO Receive5/1 -> Data Type Conversion6/1
  EtherCAT Async SDO Upload/1 -> Rate Transition/1
  Constant1/1 -> EtherCAT Async SDO Upload/1
  Rate Transition/1 -> Error Code/1
  EtherCAT Async SDO Upload/2 -> Terminator/1
  EtherCAT PDO Receive6/1 -> Data Type Conversion8/1
  Data Type Conversion8/1 -> Velocity Demand Value/1

== system atrias_system_1khz/DAQ/mtr_torque_cmd_to_medulla//elmo_signal ==
  note: Output Order:
      | rB
      | rA
      | lB
      | lA
      | rH
      | lH
  note: Input Order:
      |
      | backR
      | frontR
      | latR
      | backL
      | frontL
      | latL
  tau_cmd [Nm] x6 : Inport
  Constant10 : Constant  Value=LEG_MOTOR_CONSTANT
  Constant11 : Constant  Value=LEG_MTR_GEAR_RATIO
  Constant12 : Constant  Value=HIP_MOTOR_CONSTANT
  Constant13 : Constant  Value=HIP_MTR_GEAR_RATIO
  Constant8 : Constant  Value=MTR_HIP_MAX_CURRENT
  Constant9 : Constant  Value=MTR_MAX_COUNT
  Convert Current to Elmo PDO : Gain  Gain=1000/MTR_MAX_CONT_CURRENT
  Divide1 : Product  Inputs=*/
  Divide2 : Product  Inputs=//*
  Divide3 : Product  Inputs=//*
  Elmo Current Saturation : Saturate  UpperLimit=MTR_MAX_CURRENT  LowerLimit=-MTR_MAX_CURRENT
      settings: AttributesFormatString=Top: %<UpperLimit>\nBottom: %<LowerLimit>
  Hip Motor Current Saturation : Saturate  UpperLimit=MTR_HIP_MAX_CURRENT  LowerLimit=-MTR_HIP_MAX_CURRENT
      settings: AttributesFormatString=Top: %<UpperLimit>\nBottom: %<LowerLimit>
  Hip current limits for testing : Saturate  UpperLimit=HIP_CURRENT_LIMIT  LowerLimit=-HIP_CURRENT_LIMIT
      settings: AttributesFormatString=Top: %<UpperLimit>\nBottom: %<LowerLimit>
  LEFT_MOTOR_HIP_DIRECTION : Constant  Value=LEFT_MOTOR_HIP_DIRECTION
  LEG1_MOTOR_A_DIRECTION : Constant  Value=LEG1_MOTOR_A_DIRECTION
  LEG1_MOTOR_B_DIRECTION : Constant  Value=LEG1_MOTOR_B_DIRECTION
  LEG2_MOTOR_A_DIRECTION : Constant  Value=LEG2_MOTOR_A_DIRECTION
  LEG2_MOTOR_B_DIRECTION : Constant  Value=LEG2_MOTOR_B_DIRECTION
  Lateral Motor Saturation : Saturate  UpperLimit=HIP_MTR_MAX_TORQUE  LowerLimit=-HIP_MTR_MAX_TORQUE
      settings: AttributesFormatString=Top: %<UpperLimit>\nBottom: %<LowerLimit>
  Leg current limits for testing : Saturate  UpperLimit=LEG_CURRENT_LIMIT  LowerLimit=-LEG_CURRENT_LIMIT
      settings: AttributesFormatString=Top: %<UpperLimit>\nBottom: %<LowerLimit>
  Mux : Mux  Inputs=2
  Mux9 : Mux  Inputs=6
  Product : Product  RndMeth=Zero
  Product1 : Product  RndMeth=Zero
  RIGHT_MOTOR_HIP_DIRECTION : Constant  Value=RIGHT_MOTOR_HIP_DIRECTION
  Sagittal Motor Saturation : Saturate  UpperLimit=LEG_MTR_MAX_TORQUE  LowerLimit=-LEG_MTR_MAX_TORQUE
      settings: AttributesFormatString=Top: %<UpperLimit>\nBottom: %<LowerLimit>
  Selector : Selector  InputPortWidth=6  IndexOptions=Index vector (dialog)  Indices=[1 2 4 5 3 6]  OutputSizes=1
  Selector1 : Selector  InputPortWidth=6  IndexOptions=Index vector (dialog)  Indices=[1 2 3 4]  OutputSizes=1
  Selector2 : Selector  InputPortWidth=6  IndexOptions=Index vector (dialog)  Indices=[5 6]  OutputSizes=1
  current_cmd : Outport
  wires:
  Lateral Motor Saturation/1 -> Divide3/3
  Sagittal Motor Saturation/1 -> Divide2/3
  Convert Current to Elmo PDO/1 -> Mux/1
  Mux/1 -> Product/1
  Divide2/1 -> Elmo Current Saturation/1
  Constant12/1 -> Divide3/1
  Constant13/1 -> Divide3/2
  Constant10/1 -> Divide2/1
  Constant11/1 -> Divide2/2
  Selector2/1 -> Lateral Motor Saturation/1  "lateral"
  Selector1/1 -> Sagittal Motor Saturation/1  "sagittal"
  LEG1_MOTOR_A_DIRECTION/1 -> Mux9/1
  LEG1_MOTOR_B_DIRECTION/1 -> Mux9/2
  LEG2_MOTOR_A_DIRECTION/1 -> Mux9/3
  Mux9/1 -> Product/2
  LEG2_MOTOR_B_DIRECTION/1 -> Mux9/4
  RIGHT_MOTOR_HIP_DIRECTION/1 -> Mux9/5
  LEFT_MOTOR_HIP_DIRECTION/1 -> Mux9/6
  Product/1 -> current_cmd/1
  tau_cmd [Nm] x6/1 -> Selector/1
  Selector/1 -> Selector1/1, Selector2/1
  Hip Motor Current Saturation/1 -> Hip current limits for testing/1
  Divide3/1 -> Hip Motor Current Saturation/1
  Constant9/1 -> Divide1/1
  Constant8/1 -> Divide1/2
  Divide1/1 -> Product1/2
  Elmo Current Saturation/1 -> Leg current limits for testing/1
  Product1/1 -> Mux/2
  Hip current limits for testing/1 -> Product1/1
  Leg current limits for testing/1 -> Convert Current to Elmo PDO/1

== system atrias_system_1khz/Ramp Velocity Commands/Hold Start Time ==
  Time In : Inport  OutDataTypeStr=double
  Enable : EnablePort
  Time Out : Outport  OutDataTypeStr=double
  wires:
  Time In/1 -> Time Out/1

== system atrias_system_1khz/Start Controller/Hold Start Time ==
  Time In : Inport  OutDataTypeStr=double
  Enable : EnablePort
  Time Out : Outport  OutDataTypeStr=double
  wires:
  Time In/1 -> Time Out/1

== system atrias_system_1khz/DAQ/Drive 10/Drive state transition ==
  Status : Inport
  Bitwise Operator : simulink/Logic and Bit Operations/Bitwise Operator  logicop=AND  UseBitMask=on  BitMask=hex2dec('ff')  BitMaskRealWorld=Stored Integer
  Bitwise Operator1 : simulink/Logic and Bit Operations/Bitwise Operator  logicop=AND  UseBitMask=on  BitMask=hex2dec('80')  BitMaskRealWorld=Stored Integer
  Compare To Zero : simulink/Logic and Bit Operations/Compare To Zero  relop=~=  OutDataTypeStr=boolean
  Disable Voltage : Constant  Value=0  OutDataTypeStr=uint16
  Fault : simulink/Logic and Bit Operations/Compare To Constant  relop===  const=536  OutDataTypeStr=boolean
  Fault Reset : Constant  Value=128  OutDataTypeStr=uint16
  Fault Reset 2 : Constant  Value=128  OutDataTypeStr=uint16
  Fault reset if warning : Switch  Criteria=u2 > Threshold
  Operation enabled : simulink/Logic and Bit Operations/Compare To Constant  relop===  const=55  OutDataTypeStr=boolean
  Ready to switch ON : simulink/Logic and Bit Operations/Compare To Constant  relop===  const=49  OutDataTypeStr=boolean
  Shutdown : Constant  Value=6  OutDataTypeStr=uint16
  Switch ON : Constant  Value=7  OutDataTypeStr=uint16
  Switch ON Enable Op : Constant  Value=15  OutDataTypeStr=uint16
  Switch ON Enable Op 2 : Constant  Value=15  OutDataTypeStr=uint16
  Switch ON disabled : simulink/Logic and Bit Operations/Compare To Constant  relop===  const=80  OutDataTypeStr=boolean
  Switch{1..5} (5 alike) : Switch  Criteria=u2 > Threshold
  Switched ON : simulink/Logic and Bit Operations/Compare To Constant  relop===  const=51  OutDataTypeStr=boolean
  Control : Outport
  wires:
  Fault Reset 2/1 -> Switch5/1
  Switch5/1 -> Control/1
  Fault/1 -> Switch5/2
  Switch4/1 -> Switch5/3
  Switch ON Enable Op 2/1 -> Switch4/1
  Switch3/1 -> Switch4/3
  Operation enabled/1 -> Switch4/2
  Switch ON Enable Op/1 -> Switch3/1
  Switch2/1 -> Switch3/3
  Switched ON/1 -> Switch3/2
  Switch ON/1 -> Switch2/1
  Switch1/1 -> Switch2/3
  Ready to switch ON/1 -> Switch2/2
  Shutdown/1 -> Switch1/1
  Bitwise Operator/1 -> Switch ON disabled/1, Ready to switch ON/1, Switched ON/1, Operation enabled/1
  Fault reset if warning/1 -> Switch1/3
  Switch ON disabled/1 -> Switch1/2
  Disable Voltage/1 -> Fault reset if warning/3
  Fault Reset/1 -> Fault reset if warning/1
  Compare To Zero/1 -> Fault reset if warning/2
  Bitwise Operator1/1 -> Compare To Zero/1
  Status/1 -> Bitwise Operator/1, Bitwise Operator1/1, Fault/1

== system atrias_system_1khz/DAQ/Drive 2/Drive state transition ==
  Status : Inport
  Bitwise Operator : simulink/Logic and Bit Operations/Bitwise Operator  logicop=AND  UseBitMask=on  BitMask=hex2dec('ff')  BitMaskRealWorld=Stored Integer
  Bitwise Operator1 : simulink/Logic and Bit Operations/Bitwise Operator  logicop=AND  UseBitMask=on  BitMask=hex2dec('80')  BitMaskRealWorld=Stored Integer
  Compare To Zero : simulink/Logic and Bit Operations/Compare To Zero  relop=~=  OutDataTypeStr=boolean
  Disable Voltage : Constant  Value=0  OutDataTypeStr=uint16
  Fault : simulink/Logic and Bit Operations/Compare To Constant  relop===  const=536  OutDataTypeStr=boolean
  Fault Reset : Constant  Value=128  OutDataTypeStr=uint16
  Fault Reset 2 : Constant  Value=128  OutDataTypeStr=uint16
  Fault reset if warning : Switch  Criteria=u2 > Threshold
  Operation enabled : simulink/Logic and Bit Operations/Compare To Constant  relop===  const=55  OutDataTypeStr=boolean
  Ready to switch ON : simulink/Logic and Bit Operations/Compare To Constant  relop===  const=49  OutDataTypeStr=boolean
  Shutdown : Constant  Value=6  OutDataTypeStr=uint16
  Switch ON : Constant  Value=7  OutDataTypeStr=uint16
  Switch ON Enable Op : Constant  Value=15  OutDataTypeStr=uint16
  Switch ON Enable Op 2 : Constant  Value=15  OutDataTypeStr=uint16
  Switch ON disabled : simulink/Logic and Bit Operations/Compare To Constant  relop===  const=80  OutDataTypeStr=boolean
  Switch{1..5} (5 alike) : Switch  Criteria=u2 > Threshold
  Switched ON : simulink/Logic and Bit Operations/Compare To Constant  relop===  const=51  OutDataTypeStr=boolean
  Control : Outport
  wires:
  Fault Reset 2/1 -> Switch5/1
  Switch5/1 -> Control/1
  Fault/1 -> Switch5/2
  Switch4/1 -> Switch5/3
  Switch ON Enable Op 2/1 -> Switch4/1
  Switch3/1 -> Switch4/3
  Operation enabled/1 -> Switch4/2
  Switch ON Enable Op/1 -> Switch3/1
  Switch2/1 -> Switch3/3
  Switched ON/1 -> Switch3/2
  Switch ON/1 -> Switch2/1
  Switch1/1 -> Switch2/3
  Ready to switch ON/1 -> Switch2/2
  Shutdown/1 -> Switch1/1
  Bitwise Operator/1 -> Switch ON disabled/1, Ready to switch ON/1, Switched ON/1, Operation enabled/1
  Fault reset if warning/1 -> Switch1/3
  Switch ON disabled/1 -> Switch1/2
  Disable Voltage/1 -> Fault reset if warning/3
  Fault Reset/1 -> Fault reset if warning/1
  Compare To Zero/1 -> Fault reset if warning/2
  Bitwise Operator1/1 -> Compare To Zero/1
  Status/1 -> Bitwise Operator/1, Bitwise Operator1/1, Fault/1

== system atrias_system_1khz/DAQ/Drive 3/Drive state transition ==
  Status : Inport
  Bitwise Operator : simulink/Logic and Bit Operations/Bitwise Operator  logicop=AND  UseBitMask=on  BitMask=hex2dec('ff')  BitMaskRealWorld=Stored Integer
  Bitwise Operator1 : simulink/Logic and Bit Operations/Bitwise Operator  logicop=AND  UseBitMask=on  BitMask=hex2dec('80')  BitMaskRealWorld=Stored Integer
  Compare To Zero : simulink/Logic and Bit Operations/Compare To Zero  relop=~=  OutDataTypeStr=boolean
  Disable Voltage : Constant  Value=0  OutDataTypeStr=uint16
  Fault : simulink/Logic and Bit Operations/Compare To Constant  relop===  const=536  OutDataTypeStr=boolean
  Fault Reset : Constant  Value=128  OutDataTypeStr=uint16
  Fault Reset 2 : Constant  Value=128  OutDataTypeStr=uint16
  Fault reset if warning : Switch  Criteria=u2 > Threshold
  Operation enabled : simulink/Logic and Bit Operations/Compare To Constant  relop===  const=55  OutDataTypeStr=boolean
  Ready to switch ON : simulink/Logic and Bit Operations/Compare To Constant  relop===  const=49  OutDataTypeStr=boolean
  Shutdown : Constant  Value=6  OutDataTypeStr=uint16
  Switch ON : Constant  Value=7  OutDataTypeStr=uint16
  Switch ON Enable Op : Constant  Value=15  OutDataTypeStr=uint16
  Switch ON Enable Op 2 : Constant  Value=15  OutDataTypeStr=uint16
  Switch ON disabled : simulink/Logic and Bit Operations/Compare To Constant  relop===  const=80  OutDataTypeStr=boolean
  Switch{1..5} (5 alike) : Switch  Criteria=u2 > Threshold
  Switched ON : simulink/Logic and Bit Operations/Compare To Constant  relop===  const=51  OutDataTypeStr=boolean
  Control : Outport
  wires:
  Fault Reset 2/1 -> Switch5/1
  Switch5/1 -> Control/1
  Fault/1 -> Switch5/2
  Switch4/1 -> Switch5/3
  Switch ON Enable Op 2/1 -> Switch4/1
  Switch3/1 -> Switch4/3
  Operation enabled/1 -> Switch4/2
  Switch ON Enable Op/1 -> Switch3/1
  Switch2/1 -> Switch3/3
  Switched ON/1 -> Switch3/2
  Switch ON/1 -> Switch2/1
  Switch1/1 -> Switch2/3
  Ready to switch ON/1 -> Switch2/2
  Shutdown/1 -> Switch1/1
  Bitwise Operator/1 -> Switch ON disabled/1, Ready to switch ON/1, Switched ON/1, Operation enabled/1
  Fault reset if warning/1 -> Switch1/3
  Switch ON disabled/1 -> Switch1/2
  Disable Voltage/1 -> Fault reset if warning/3
  Fault Reset/1 -> Fault reset if warning/1
  Compare To Zero/1 -> Fault reset if warning/2
  Bitwise Operator1/1 -> Compare To Zero/1
  Status/1 -> Bitwise Operator/1, Bitwise Operator1/1, Fault/1

== system atrias_system_1khz/DAQ/Drive 9/Drive state transition ==
  Status : Inport
  Bitwise Operator : simulink/Logic and Bit Operations/Bitwise Operator  logicop=AND  UseBitMask=on  BitMask=hex2dec('ff')  BitMaskRealWorld=Stored Integer
  Bitwise Operator1 : simulink/Logic and Bit Operations/Bitwise Operator  logicop=AND  UseBitMask=on  BitMask=hex2dec('80')  BitMaskRealWorld=Stored Integer
  Compare To Zero : simulink/Logic and Bit Operations/Compare To Zero  relop=~=  OutDataTypeStr=boolean
  Disable Voltage : Constant  Value=0  OutDataTypeStr=uint16
  Fault : simulink/Logic and Bit Operations/Compare To Constant  relop===  const=536  OutDataTypeStr=boolean
  Fault Reset : Constant  Value=128  OutDataTypeStr=uint16
  Fault Reset 2 : Constant  Value=128  OutDataTypeStr=uint16
  Fault reset if warning : Switch  Criteria=u2 > Threshold
  Operation enabled : simulink/Logic and Bit Operations/Compare To Constant  relop===  const=55  OutDataTypeStr=boolean
  Ready to switch ON : simulink/Logic and Bit Operations/Compare To Constant  relop===  const=49  OutDataTypeStr=boolean
  Shutdown : Constant  Value=6  OutDataTypeStr=uint16
  Switch ON : Constant  Value=7  OutDataTypeStr=uint16
  Switch ON Enable Op : Constant  Value=15  OutDataTypeStr=uint16
  Switch ON Enable Op 2 : Constant  Value=15  OutDataTypeStr=uint16
  Switch ON disabled : simulink/Logic and Bit Operations/Compare To Constant  relop===  const=80  OutDataTypeStr=boolean
  Switch{1..5} (5 alike) : Switch  Criteria=u2 > Threshold
  Switched ON : simulink/Logic and Bit Operations/Compare To Constant  relop===  const=51  OutDataTypeStr=boolean
  Control : Outport
  wires:
  Fault Reset 2/1 -> Switch5/1
  Switch5/1 -> Control/1
  Fault/1 -> Switch5/2
  Switch4/1 -> Switch5/3
  Switch ON Enable Op 2/1 -> Switch4/1
  Switch3/1 -> Switch4/3
  Operation enabled/1 -> Switch4/2
  Switch ON Enable Op/1 -> Switch3/1
  Switch2/1 -> Switch3/3
  Switched ON/1 -> Switch3/2
  Switch ON/1 -> Switch2/1
  Switch1/1 -> Switch2/3
  Ready to switch ON/1 -> Switch2/2
  Shutdown/1 -> Switch1/1
  Bitwise Operator/1 -> Switch ON disabled/1, Ready to switch ON/1, Switched ON/1, Operation enabled/1
  Fault reset if warning/1 -> Switch1/3
  Switch ON disabled/1 -> Switch1/2
  Disable Voltage/1 -> Fault reset if warning/3
  Fault Reset/1 -> Fault reset if warning/1
  Compare To Zero/1 -> Fault reset if warning/2
  Bitwise Operator1/1 -> Compare To Zero/1
  Status/1 -> Bitwise Operator/1, Bitwise Operator1/1, Fault/1

== matlab function atrias_system_1khz/DAQ/logic_voltage_volts ==
  data: u input; volt output; MEDULLA_ADC_OFFSET_COUNTS parameter; MEDULLA_ADC_MAX_VOLTS parameter
function volt = fcn(u, MEDULLA_ADC_OFFSET_COUNTS, MEDULLA_ADC_MAX_VOLTS)
% Taken from Medulla.cpp in the ATRIAS medulla drivers
% at code.google.com/p/atrias
adcReadingVolts = (u - MEDULLA_ADC_OFFSET_COUNTS) * MEDULLA_ADC_MAX_VOLTS/4095;
volt            = 6 * adcReadingVolts;

== matlab function atrias_system_1khz/DAQ/medulla_errors ==
  data: u input; errors output
function errors = fcn(u)
% right back, right front, left back, left front, left lateral, right lateral, boom
errors = reshape(bsxfun(@bitand,u,2.^[0 1 2 3 4 5 6 7]),[],1);

== matlab function atrias_system_1khz/Compute State Command ==
  data: medulla_states input uint8; elmo_enable output; medulla_cmd output; should_estop input boolean; should_halt input boolean; gui_enable_cmd parameter boolean; gui_disable_cmd parameter boolean; gui_reset_cmd parameter boolean; gui_exit_cmd parameter boolean; MEDULLA_STATE_IDLE parameter uint8; MEDULLA_STATE_RUN parameter uint8; MEDULLA_STATE_HALT parameter uint8; MEDULLA_STATE_ERROR parameter uint8; MEDULLA_STATE_RESET parameter uint8; any_halt output boolean; stop_model output
function [elmo_enable,medulla_cmd,any_halt,stop_model] = fcn(medulla_states,      ...
                                                             should_estop,        ...
                                                             should_halt,         ...
                                                             gui_enable_cmd,      ...
                                                             gui_disable_cmd,     ...
                                                             gui_reset_cmd,       ...
                                                             gui_exit_cmd,        ...
                                                             MEDULLA_STATE_IDLE,  ...
                                                             MEDULLA_STATE_RUN,   ...
                                                             MEDULLA_STATE_HALT,  ...
                                                             MEDULLA_STATE_ERROR, ...
                                                             MEDULLA_STATE_RESET)
%#codegen

% Count the number of medullas in each state
any_idle  = any(medulla_states == MEDULLA_STATE_IDLE );
any_reset = any(medulla_states == MEDULLA_STATE_RESET);
any_run   = any(medulla_states == MEDULLA_STATE_RUN  );
any_halt  = any(medulla_states == MEDULLA_STATE_HALT );
any_estop = any(medulla_states == MEDULLA_STATE_ERROR);

% Except in one case, we don't want to stop the model
stop_model = false;

% Special-case for if the GUI is commanding a model stop
if gui_exit_cmd
    % We always want to disable the amplifiers if a stop is commanded
    elmo_enable = false;

    % Stop a currently in-progress halt. if one is occurring.
    % This may only be done with an estop
    if any_halt
        medulla_cmd = MEDULLA_STATE_ERROR;
        return
    end

    % If an estop has occurred, reset the medullas
    if any_estop
        medulla_cmd = MEDULLA_STATE_RESET;
        return
    end

    % At this point, there are no error states, so command idle
    medulla_cmd = MEDULLA_STATE_IDLE;

    % If all medullas have entered idle (we've already checked halt and
    % estop), then stop the model
    if ~any_reset && ~any_run
        stop_model = true;
    end

    % Unconditionally quit here to the remainder of the logic does not run
    return
end

% Compute whether or not to reset based on the current states and the
% GUI's input
should_reset = gui_reset_cmd  && ...
              ~gui_enable_cmd && ... % Make sure we're not about to re-enable (precaution)
               any_estop      && ... % A medulla must be e-stopped (precaution)
              ~any_halt       && ... % No medullas may be halting (precaution)
              ~any_run;              % No medullas may be running (precaution)

% Send an E-Stop first if the safeties are engaging, so this can't fail.
% Also send an E-Stop if any medullas are E-stopped, unless the GUI is
% sending a reset command
if ((any_run || any_halt) && should_estop) || (any_estop && ~should_reset)
    elmo_enable = false;
    medulla_cmd = MEDULLA_STATE_ERROR;
    return
end

% If any Medullas are halting, automatically command halt for all.
% If we want to command a halt while we're in run, command a halt.
if any_halt || (any_run && should_halt)
    elmo_enable = true;
    medulla_cmd = MEDULLA_STATE_HALT;
    return
end

% Allow for GUI-commanded resets. Make sure an enable command isn't being
% sent as an enable precaution
if should_reset || any_reset
    elmo_enable = false;
    medulla_cmd = MEDULLA_STATE_RESET;
    return
end

% Past this point, the robot should be either enabled or disabled
% (no E-Stops or halts)

% Allow the GUI to disable the robot.
% For now, there is no soft shutdown.
if gui_disable_cmd
    elmo_enable = false;
    medulla_cmd = MEDULLA_STATE_IDLE;
    return
end

% Allow for enabling (when safeties aren't triggered)
if gui_enable_cmd && ~should_estop && ~should_halt
    elmo_enable = true;
    medulla_cmd = MEDULLA_STATE_RUN;
    return
end

% Since we have no errors or relevant GUI commands, just mimic the
% Medullas's current states
if any_idle
    elmo_enable = false;
    medulla_cmd = MEDULLA_STATE_IDLE;
    return
else
    elmo_enable = true;
    medulla_cmd = MEDULLA_STATE_RUN;
    return
end
end

== matlab function atrias_system_1khz/DAQ/motor_temperatures ==
  data: u input; temp output
function temp = fcn(u)
adc_values = ((u - 172.0) * (2.70/(4095.0)));
temp = ((1.0./( (1.0/298.15) + (1.0/3988.0)*log(4700.0./((3.26./adc_values) - 1.0)/10000))) - 273.15);

== matlab function atrias_system_1khz/DAQ/motor_voltage_volts ==
  data: u input; volt output
function volt = fcn(u)
% 1300 counts = 0 V
volt = (u - 1300.0) * 60.2 / (3600.0 - 1300.0);

== matlab function atrias_system_1khz/Latch Diagnostics ==
  data: reset input boolean; diags input boolean; diags_out output uint8
function diags_out = fcn(reset, diags)
%#codegen

% Recall the values of our diagnostics through a persistent variable.
% We are using a persistent variable to allow the vector to be resized
% automatically to fit the size of diags
persistent latchedDiags

% Initialize latchedDiags
if isempty(latchedDiags)
    latchedDiags = uint8(zeros(numel(diags), 1));
end


% If we're idle, then reset the counter and forward the diagnostics
% directly through.
if reset
    latchedDiags = uint8(diags);
    diags_out    = uint8(diags);
    return
end

% Since we're not idle, Sequence the diagnostics and latch the
% results    
updates    = diags & (~logical(latchedDiags));
newCounter = max(latchedDiags);
% Protect against counter overflow
if newCounter + 1 > newCounter
    newCounter = newCounter + 1;
end

% Perform the update of newly-activated diagnostic events
latchedDiags(updates) = newCounter;
diags_out             = latchedDiags;

== matlab function atrias_system_1khz/DAQ/Limit Switches to Bool ==
  data: sw input; sw_out output boolean
function sw_out  = fcn(sw)
%#codegen

% Binary decode (split the input into an array of booleans)
% This creates a matrix; each column corresponds with one of the original
% input uint8's, and each row corresponds with a bit location within the
% octet.
sw = bsxfun(@bitand, uint8(2.^(0:7)), uint8(sw(2:2:end)))';

% Reshape and cast our output to make Simulink happy
sw_out = logical(sw(:));

== matlab function atrias_system_1khz/Mux Diags ==
  data: Halting input; diags output boolean; SW input; ErrorFlags input uint8; ControllerFault input boolean; softLimits input; decelFailEstop input; transmissionLimits input
function diags = fcn(Halting, SW, ErrorFlags, ControllerFault, softLimits, decelFailEstop, transmissionLimits)
%#codegen

% Convert error flags into a boolean array.
% This will generate one column per medulla and one row per bit,
% so when we read it into diags later on it will come out in the right
% order.
ErrorFlags = logical(bsxfun(@bitand, uint8(2.^(0:7)), ErrorFlags))';

% Generate diags from the processed inputs
diags = [ Halting
          SW
          ErrorFlags(:)
          ControllerFault
          softLimits
          decelFailEstop
          transmissionLimits];
